simulink model "sf_varsize_example"  (Simulink 7.6)
settings: Solver=FixedStepDiscrete  StartTime=0.0  StopTime=inf  FixedStep=0.05  RelTol=1e-3
settings Model: Creator=The MathWorks Inc.
settings DebuggingCC: StrictBusMsg=Warning
settings SFSimCC: SimParseCustomCode=off

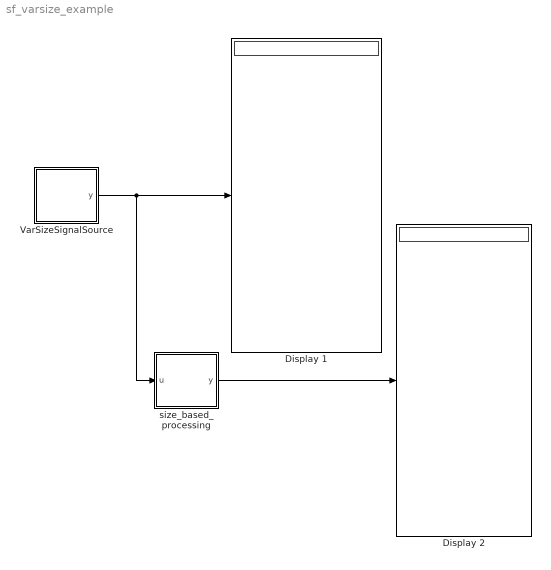
== system sf_varsize_example ==
  Display 1 : Display
  Display 2 : Display
  VarSizeSignalSource : Stateflow chart  TreatAsAtomicUnit=on
  size_based_processing : Stateflow chart  TreatAsAtomicUnit=on
  wires:
  VarSizeSignalSource/1(y) -> Display 1/1, size_based_processing/1(u)
  size_based_processing/1(y) -> Display 2/1

== stateflow chart VarSizeSignalSource ==
  state Scalar
    en: generateOutput(1);
    du: generateOutput(1);
  state VectorPartial
    en: generateOutput(8);
    du: generateOutput(8);
  state VectorFull
    en: generateOutput(16);
    du: generateOutput(16);
  note: Use this Stateflow chart to generate an output signal with a variable size.  In this chart,
      | each state calls an Embedded MATLAB function that assigns to the chart output
      | a different-sized signal (within the bounds).  During simulation, transitions between states
      | change the size of the signal. You can use this variable-size signal to test other blocks
      | and subsystems in your model.
  (default) -> Scalar
  Scalar -> VectorPartial : [after(5,tick)]
  VectorPartial -> VectorFull : [after(5,tick)]
  VectorFull -> Scalar : [after(5,tick)]
  data: len function_input double; y output double size=16
  function generateOutput(len):
    | function generateOutput(len)
    | %#eml
    | assert(len<=16);
    | y = (1:len)';

== stateflow chart size_based_processing ==
  note: In this chart, Embedded MATLAB functions:
      | (a) Determine the size of the input signal.
      | (b) Use MATLAB syntax to compute variable-size outputs based on inputs.
      | (c) Reset the output to zero when the input is scalar.
      |
      | Key behavior:
      | 1. Variable-size data are allowed only for chart input and output data.
      | 2. Variable-size data "u" and "y" do not appear in state actions or on transitions.
      | 3. Embedded MATLAB functions access variable-size data "u" and y" directly for computations.
      | 4. Embedded MATLAB functions do not use variable dimensions for their own input and output data.
  state Scalar
    reset_output();
  state Vector
    en: compute_output();
    du: compute_output();
  (default) -> Scalar
  Scalar -> Vector : [!is_scalar_input()]
  Vector -> Scalar : [is_scalar_input()]
  data: isScalar function_output boolean; u input double size=16; y output double size=16
  function isScalar = is_scalar_input:
    | function isScalar = is_scalar_input
    | %#eml
    | isScalar = length(u)==1;
  function reset_output:
    | function reset_output
    | %#eml
    | y = 0;
  function compute_output:
    | function compute_output
    | %#eml
    | y = sin(u);
